simulink model "rlc_simulink"  (R2015a)
settings: Solver=ode45  StartTime=0.0  StopTime=10.0  RelTol=1e-3
undefined symbols (not defined in the file): C, L, R, Vin
settings Model: Creator=sseshadr  LastModifiedBy=sseshadr

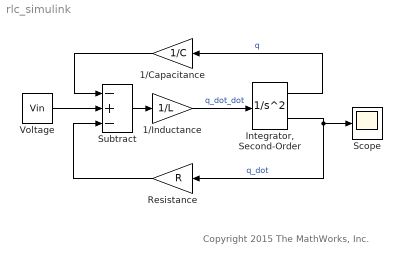
== system rlc_simulink ==
  note: Copyright 2015 The MathWorks, Inc.
  1/Capacitance : Gain  Gain=1/C
  1/Inductance : Gain  Gain=1/L
  "Integrator, Second-Order" : SecondOrderIntegrator
  Resistance : Gain  Gain=R
  Scope : Scope
  Subtract : Sum  Inputs=-+-
  Voltage : Constant  Value=Vin
  wires:
  Subtract/1 -> 1/Inductance/1
  "Integrator, Second-Order"/1 -> 1/Capacitance/1  "q"
  1/Inductance/1 -> "Integrator, Second-Order"/1  "q_dot_dot"
  Voltage/1 -> Subtract/2
  1/Capacitance/1 -> Subtract/1
  "Integrator, Second-Order"/2 -> Scope/1, Resistance/1  "q_dot"
  Resistance/1 -> Subtract/3
